simulink model "DirectMRAC"  (R2019b)
settings: Solver=VariableStepAuto  StartTime=0.0  StopTime=10.0  RelTol=1e-3
values from neighbouring files (symbols this model uses):
  a = 15    [directmrac workspace.mat]    (also in lin_state_estimator.mat = [-3  -4; 2  1])
  am = 10    [directmrac workspace.mat]
  b = 20    [directmrac workspace.mat]    (also in lin_state_estimator.mat = [1 0]; online_estimator.mat = [1 2.2])
  bm = 1    [directmrac workspace.mat]
  ep = 0.001    [directmrac workspace.mat]
  gam = 2    [directmrac workspace.mat]
libraries: simulink x1
settings Model: Creator=chint  LastModifiedBy=chint

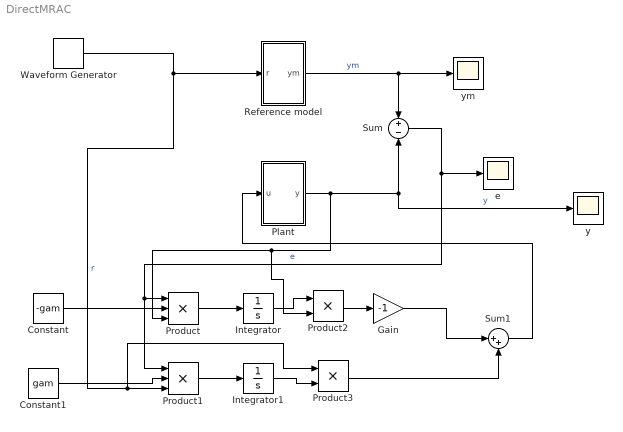
== system DirectMRAC ==
  Constant : Constant  Value=-gam
  Constant1 : Constant  Value=gam
  Gain : Gain  Gain=-1
  Integrator : Integrator
  Integrator1 : Integrator
  Plant : Subsystem
  Product : Product  Inputs=3
  Product1 : Product  Inputs=3
  Product2 : Product
  Product3 : Product
  Reference model : Subsystem
  Sum : Sum  Inputs=+-
  Sum1 : Sum  Inputs=|++
  Waveform Generator : simulink/Sources/Waveform Generator  OutMin=[]  OutMax=[]  OutDataTypeStr=double  SelectedSignal=1  Signals=sin(2,3,1)  BlockNames=MultiportSwitch_458b37d82ce1408  SampleTime=0.1
      settings: SourceProductName=Simulink
  e : Scope
  y : Scope
  ym : Scope
  wires:
  Waveform Generator/1 -> Product3/1, Product1/3, Reference model/1(r)  "r"
  Reference model/1(ym) -> ym/1, Sum/1  "ym"
  Plant/1(y) -> Product2/2, Product/3, Sum/2, y/1  "y"
  Sum/1 -> e/1, Product1/1, Product/1  "e"
  Constant/1 -> Product/2
  Constant1/1 -> Product1/2
  Product/1 -> Integrator/1
  Product1/1 -> Integrator1/1
  Integrator/1 -> Product2/1
  Integrator1/1 -> Product3/2
  Product2/1 -> Gain/1
  Gain/1 -> Sum1/1
  Product3/1 -> Sum1/2
  Sum1/1 -> Plant/1(u)

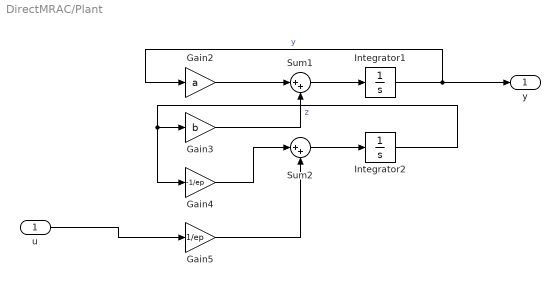
== system DirectMRAC/Plant ==
  u : Inport
  Gain2 : Gain  Gain=a
  Gain3 : Gain  Gain=b
  Gain4 : Gain  Gain=-1/ep
  Gain5 : Gain  Gain=1/ep
  Integrator1 : Integrator
  Integrator2 : Integrator
  Sum1 : Sum  Inputs=|++
  Sum2 : Sum  Inputs=|++
  y : Outport
  wires:
  Gain3/1 -> Sum1/2
  Integrator2/1 -> Gain4/1, Gain3/1  "z"
  Gain5/1 -> Sum2/2
  u/1 -> Gain5/1
  Integrator1/1 -> y/1, Gain2/1  "y"
  Sum1/1 -> Integrator1/1
  Sum2/1 -> Integrator2/1
  Gain2/1 -> Sum1/1
  Gain4/1 -> Sum2/1

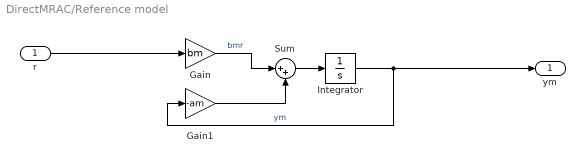
== system DirectMRAC/Reference model ==
  r : Inport
  Gain : Gain  Gain=bm
  Gain1 : Gain  Gain=-am
  Integrator : Integrator
  Sum : Sum  Inputs=|++
  ym : Outport
  wires:
  Gain/1 -> Sum/1  "bmr"
  Integrator/1 -> ym/1, Gain1/1  "ym"
  Sum/1 -> Integrator/1
  r/1 -> Gain/1
  Gain1/1 -> Sum/2
